simulink model "TestA__03"  (R2015b)
settings: Solver=ode23tb  StartTime=0.0  StopTime=.3  RelTol=1e-3
PreLoadFcn:
  | t1=1;
InitFcn:
  | t_Pref1=0.09; Pref1=10e2;
  | t_Pref2=0.3;   Pref2=3e5;
  | 
  | t_Qmax1=.12; t_Qmax2=t_Qmax1+.01;
  | t_Qref1=0.09; Qref1=7e5;
  | t_Qref2=0.5; Qref2=10e5;
  | 
  | t_Imax1=.2; Imax1=1200;
  | t_Imax2=.4; Imax2=1500;
  | 
  | t_k1=0.25; k1=.8;
  | t_k2=0.35; k2=.2;
  | t_h1=0.45; h1=.9;
  | t_h2=0.55; h2=.5;
  | 
  | Lg=90e-6;
  | l=100e-6; r=2e-3;
  | tff=10e-6;
  | w=2*pi*60;
  | z_lead =966.3602;
  | p_lead =5.6324e+03;
  | Vdc=10000;
  | Vs=690;
undefined symbols (not defined in the file or in its folder): magnitude
libraries: powerlib x43, powerlib_meascontrol x10, simulink x4, simulink_extras x3
settings Model: Creator=Shahed Mortazavian  LastModifiedBy=Masoud
settings DataIOCC: SaveFormat=Array  SignalLoggingSaveFormat=ModelDataLogs
settings OptimizationCC: ExpressionDepthLimit=2147483647
settings DebuggingCC: UnderspecifiedInitializationDetection=Classic  MergeDetectMultiDrivingBlocksExec=none  SolverPrmCheckMsg=warning  FcnCallInpInsideContextMsg=UseLocalSettings  StateNameClashWarn=warning
settings HardwareCC: ProdBitPerPointer=32  ProdLargestAtomicFloat=None  ProdIntDivRoundTo=Undefined  ProdEndianess=Unspecified  ProdWordSize=32  ProdHWDeviceType=32-bit Generic
settings GRTTargetCC: GeneratePreprocessorConditionals=Disable all  CombineOutputUpdateFcns=off  GRTInterface=on
settings ConfigComp: CovModelRefEnable=Off  CovSFcnEnable=off

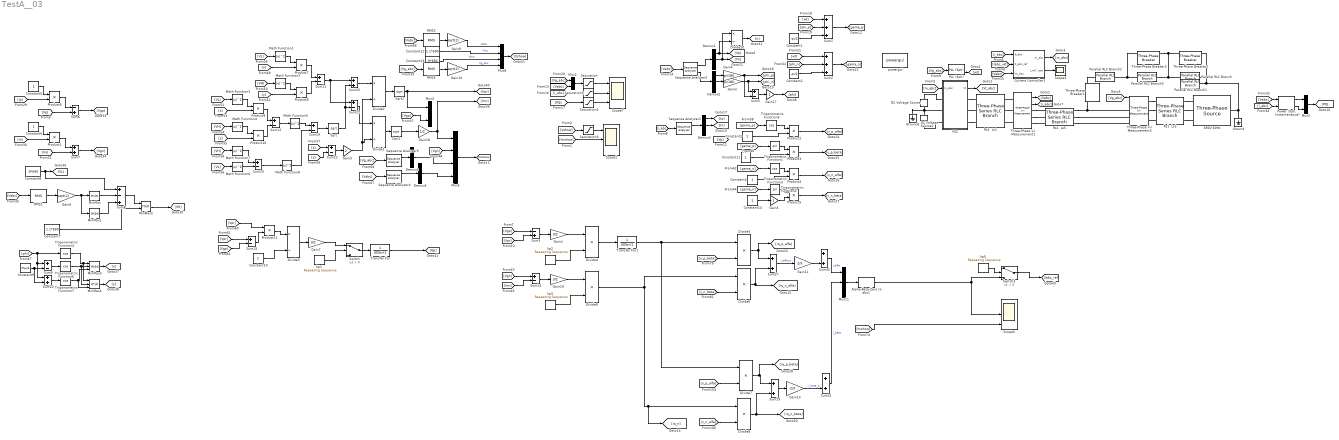
== system TestA__03 ==
  690V 60Hz : powerlib/Electrical Sources/Three-Phase Source  InternalConnection=Yn  VoltagePhases=off  Voltage=Vs*sqrt(3)/sqrt(2)  PhaseAngle=0  Voltage_phases=[25e3 25e3 25e3]/sqrt(3)  PhaseAngles_phases=[0 -120 +120]  Frequency=60  NonIdealSource=on  SpecifyImpedance=off  Resistance=2e-10  Inductance=1e-10  ShortCircuitLevel=100e6  BaseVoltage=25e3  XRratio=7  BusType=swing  Pref=0  Qref=0  Prefabc=[10e3, 10e3, 10e3]  Qrefabc=[0, 0, 0]  Qmin=-inf  Qmax=inf
  Alpha-Beta-Zero to abc1 : powerlib_meascontrol/Transformations/Alpha-Beta-Zero to abc
  Constant1 : Constant  Value=-pi/2
  Constant{3..6,10..11,14} (7 alike) : Constant
  Constant12 : Constant  Value=1.1*690
  Constant13 : Constant  Value=.9*690
  Constant2 : Constant  Value=-pi/2
  Constant7 : Constant  Value=1.1*690
  Constant8 : Constant  Value=.9*690
  Constant9 : Constant  Value=2*pi/3
  Current Controller1 : Subsystem
  DC Voltage Source : powerlib/Electrical Sources/DC Voltage Source  Amplitude=Vdc/2  Measurements=None
  DC Voltage Source1 : powerlib/Electrical Sources/DC Voltage Source  Amplitude=Vdc/2  Measurements=None
  Demux{1..5} (5 alike) : Demux  Outputs=3
  Divide{1..3,20} (4 alike) : Product  Inputs=*/
  Divide{4..9} (6 alike) : Product  Inputs=**
  Gain1 : Gain  Gain=3/2
  Gain10 : Gain  Gain=-2/3
  Gain11 : Gain  Gain=2/3
  Gain16 : Gain  Gain=sqrt(2)
  Gain17 : Gain
  Gain18 : Gain  Gain=1/2
  Gain19 : Gain  Gain=3/2
  Gain2 : Gain  Gain=pi/180
  Gain3 : Gain  Gain=2
  Gain4 : Gain  Gain=pi/180
  Gain5 : Gain  Gain=-1
  Gain6 : Gain  Gain=sqrt(2)
  Gain7 : Gain  Gain=3/2
  Gain9 : Gain  Gain=sqrt(2)
  Ground : powerlib/Elements/Ground  LConnTagsString=a
  Ground1 : powerlib/Elements/Ground  LConnTagsString=a
  Math Function{1..8} (8 alike) : Math  Operator=magnitude^2  SaturateOnIntegerOverflow=on
  MinMax : MinMax
  MinMax1 : MinMax  Function=max
  MinMax2 : MinMax  Inputs=2
  MinMax3 : MinMax  Function=max  Inputs=3
  MinMax4 : MinMax  Inputs=3
  Mux11 : Mux  Inputs=3
  Mux2 : Mux  Inputs=2
  Mux3 : Mux  Inputs=2
  Mux4 : Mux  Inputs=2
  Mux5 : Mux
  Mux8 : Mux
  PLL (3ph) : powerlib_meascontrol/PLL/PLL (3ph)  Fmin=45  Par_Init=[0, 60]  ParK=[180, 3200, 1]  TcD=1e-4  MaxRateChangeFreq=12  FilterCutOffFreq=25  Ts=0  AGC=on
  Parallel RLC Branch : powerlib/Elements/Parallel RLC Branch  LConnTagsString=a  RConnTagsString=__new0  BranchType=R  Resistance=2e-3  Inductance=1e-3  SetiL0=off  InitialCurrent=0  Capacitance=1e-6  Setx0=off  InitialVoltage=0  Measurements=None
  Parallel RLC Branch1 : powerlib/Elements/Parallel RLC Branch  LConnTagsString=a  RConnTagsString=__new0  BranchType=R  Resistance=.02  Inductance=1e-3  SetiL0=off  InitialCurrent=0  Capacitance=1e-6  Setx0=off  InitialVoltage=0  Measurements=None
  Parallel RLC Branch2 : powerlib/Elements/Parallel RLC Branch  LConnTagsString=a  RConnTagsString=__new0  BranchType=R  Resistance=3e-3  Inductance=1e-3  SetiL0=off  InitialCurrent=0  Capacitance=1e-6  Setx0=off  InitialVoltage=0  Measurements=None
  Parallel RLC Branch3 : powerlib/Elements/Parallel RLC Branch  LConnTagsString=a  RConnTagsString=__new0  BranchType=R  Resistance=1e-3  Inductance=1e-3  SetiL0=off  InitialCurrent=0  Capacitance=1e-6  Setx0=off  InitialVoltage=0  Measurements=None
  "Power (3ph, Instantaneous)" : powerlib_meascontrol/Measurements/Power (3ph, Instantaneous)
  Product{1..11} (11 alike) : Product
  RMS1 : powerlib_meascontrol/Measurements/RMS  TrueRMS=on  Freq=60  RMSInit=0  Ts=0
  RMS2 : powerlib_meascontrol/Measurements/RMS  TrueRMS=on  Freq=60  RMSInit=0  Ts=0
  RMS5 : powerlib_meascontrol/Measurements/RMS  TrueRMS=on  Freq=60  RMSInit=0  Ts=0
  Rs1  Ls1 : powerlib/Elements/Three-Phase Series RLC Branch  LConnTagsString=A|B|C  RConnTagsString=A|B|C  BranchType=RL  Resistance=r  Inductance=l  Capacitance=1e-6  Measurements=None
  Rs1  Ls2 : powerlib/Elements/Three-Phase Series RLC Branch  LConnTagsString=A|B|C  RConnTagsString=A|B|C  BranchType=R  Resistance=1e-3  Inductance=l  Capacitance=1e-6  Measurements=None
  Rs1  Ls5 : powerlib/Elements/Three-Phase Series RLC Branch  LConnTagsString=A|B|C  RConnTagsString=A|B|C  BranchType=RL  Resistance=1e-3  Inductance=1/377  Capacitance=1e-6  Measurements=None
  Saturation : Saturate  UpperLimit=1000  LowerLimit=-1000
  Saturation1 : Saturate  UpperLimit=200  LowerLimit=-200
  Saturation2 : Saturate  UpperLimit=2e5  LowerLimit=-1e5
  Saturation3 : Saturate  UpperLimit=800  LowerLimit=400
  Scope2 : Scope  NumInputPorts=3
  Scope3 : Scope
  Scope5 : Scope  NumInputPorts=3
  Scope7 : Scope  NumInputPorts=3
  Sequence Analyzer{1..4} (4 alike) : powerlib_meascontrol/Measurements/Sequence Analyzer  Freq=60  n=1  seq=Positive Negative Zero  InInit=[1, 0]  Ts=0
  Sqrt : Sqrt  SaturateOnIntegerOverflow=on
  Sqrt1 : Sqrt  SaturateOnIntegerOverflow=on
  Sqrt2 : Sqrt  SaturateOnIntegerOverflow=on
  Sum1 : Sum  Inputs=+++
  Sum{7,10,23,27,29..31} (7 alike) : Sum
  Sum{5,9,11..12,14,19..22,24} (10 alike) : Sum  Inputs=+-
  Sum2 : Sum  Inputs=+++
  Sum3 : Sum  Inputs=-+
  Sum6 : Sum  Inputs=-+
  Sum8 : Sum  Inputs=+-+
  Switch : Switch  Criteria=u2 > Threshold
  Switch3 : Switch  Criteria=u2 > Threshold
  Three-Phase V-I Measurement1 : powerlib/Measurements/Three-Phase V-I Measurement  VoltageMeasurement=phase-to-ground  SetLabelV=off  LabelV=Vabc  Vpu=off  VpuLL=off  CurrentMeasurement=yes  SetLabelI=off  LabelI=Iabc  Ipu=off  Pbase=100e6  Vbase=500e3  OutputType=Complex  PhasorSimulation=off  PSBequivalent=0
  Three-Phase V-I Measurement3 : powerlib/Measurements/Three-Phase V-I Measurement  VoltageMeasurement=phase-to-ground  SetLabelV=off  LabelV=Vabc  Vpu=off  VpuLL=off  CurrentMeasurement=yes  SetLabelI=off  LabelI=Iabc  Ipu=off  Pbase=100e6  Vbase=500e3  OutputType=Complex  PhasorSimulation=off  PSBequivalent=0
  Three-Phase Breaker1 : powerlib/Elements/Three-Phase Breaker  InitialState=open  SwitchA=on  SwitchB=on  SwitchC=on  SwitchTimes=[.05 10]  External=off  BreakerResistance=1e-40  SnubberResistance=1e6  SnubberCapacitance=inf  Measurements=None
  Three-Phase Breaker2 : powerlib/Elements/Three-Phase Breaker  InitialState=open  SwitchA=on  SwitchB=on  SwitchC=on  SwitchTimes=.1  External=off  BreakerResistance=1e-40  SnubberResistance=1e6  SnubberCapacitance=inf  Measurements=None
  Three-Phase Breaker3 : powerlib/Elements/Three-Phase Breaker  InitialState=open  SwitchA=on  SwitchB=on  SwitchC=on  SwitchTimes=.15  External=off  BreakerResistance=1e-40  SnubberResistance=1e6  SnubberCapacitance=inf  Measurements=None
  Transfer Fcn : TransferFcn  Denominator=[.005 1]
  Transfer Fcn1 : TransferFcn  Denominator=[.005 1]
  Trigonometric Function1 : Trigonometry
  Trigonometric Function2 : Trigonometry
  Trigonometric Function{3..7} (5 alike) : Trigonometry  Operator=cos
  VSC : Subsystem
  kp1 : simulink/Sources/Repeating Sequence  rep_seq_t=[0 .055 .055+eps 10]  rep_seq_y=[0 0 1 1]
  kp2 : simulink/Sources/Repeating Sequence  rep_seq_t=[0 .055 .055+eps 10]  rep_seq_y=[0 0 1 1]
  kp3 : simulink/Sources/Repeating Sequence  rep_seq_t=[0 .2 .2+eps 10]  rep_seq_y=[0 0 1 1]
  kp5 : simulink/Sources/Repeating Sequence  rep_seq_t=[0 .6 .6+eps 10]  rep_seq_y=[0 0 1 1]
  powergui : powerlib/powergui  Priority=2  SimulationMode=Discrete  SolverType=Tustin  SampleTime=5e-5  frequency=60  SPID=off  DisableSnubberDevices=off  DisableRonSwitches=off  DisableVfSwitches=off  SwTol=0  DisplayEquations=off  Interpol=off  ExternalGateDelay=off  methode=off  Ts=0  FunctionMessages=off  echomessages=off  HookPort=off  EnableUseOfTLC=off  x0status=blocks  frequencyindice=0  Pbase=100e6  ErrMax=1e-4  Iterations=50  UnitsV=kV  UnitsW=MW  buscounter=0  RestoreLinks=warning  ResistiveCurrentMeasurement=off  Frange=[0:2:500]  Ylog=off  Xlog=on  ShowGrid=off  save=off  variable=ZData  structure=Data  ZoomFFT=off  StartTime=.22  cycles=2  DisplayStyle=1  fundamental=60  FreqAxis=off  MaxFrequency=1000  frequencyindicesteady=1  RmsSteady=1  display=off
  wires:
  Three-Phase V-I Measurement1/1 -> [Vabc]
  VSC/1(Vt) -> [Vt_abc]
  [m_abc] -> VSC/1(m_abc)
  Three-Phase V-I Measurement3/1 -> [Vg_abc]
  Three-Phase V-I Measurement1/2 -> [i_abc]
  [Vabc] -> Sequence Analyzer2/1
  [i_abc] -> Current Controller1/1(It_abc)
  [Vabc] -> Current Controller1/3(Vs_abc)
  Current Controller1/1(m_abc) -> [m_abc]
  [Iabc_ref] -> Current Controller1/2(It_abc_ref)
  [Vg_abc] -> PLL (3ph)/1
  PLL (3ph)/2 -> [wt]
  [i_abc] -> Saturation1/1
  [PQ] -> Saturation2/1
  Mux2/1 -> Saturation/1
  [Vabc] -> Mux2/2
  [Vg_abc] -> Mux2/1
  Sequence Analyzer2/1 -> Demux1/1
  Demux1/1 -> Divide20/2, [Vp]
  Demux2/1 -> Gain4/1
  Sequence Analyzer2/2 -> Demux2/1
  Demux2/2 -> Gain2/1
  Demux1/2 -> Divide20/1, [Vn]
  "Power (3ph, Instantaneous)"/1 -> Mux3/1
  "Power (3ph, Instantaneous)"/2 -> Mux3/2
  [Vabc] -> "Power (3ph, Instantaneous)"/1
  [i_abc] -> "Power (3ph, Instantaneous)"/2
  Mux3/1 -> [PQ]
  Gain4/1 -> [phi_p], Sum5/2
  Gain2/1 -> [phi_n], Sum5/1
  [gama_p] -> Trigonometric Function5/1
  Trigonometric Function5/1 -> Product2/1
  Constant3/1 -> Product2/2
  [gama_p] -> Trigonometric Function1/1
  Trigonometric Function1/1 -> Product3/1
  [gama_n] -> Trigonometric Function3/1
  Trigonometric Function3/1 -> Product4/1
  Product4/1 -> [v_n_alfa]
  [gama_n] -> Trigonometric Function2/1
  Trigonometric Function2/1 -> Product5/1
  Product5/1 -> [v_n_beta]
  Constant14/1 -> Gain5/1
  Constant4/1 -> Product4/2
  Gain5/1 -> Product5/2
  Product2/1 -> [v_p_alfa]
  Product3/1 -> [v_p_beta]
  Constant11/1 -> Product3/2
  Sum5/1 -> Gain17/1
  [Vp] -> Sum6/2
  Constant5/1 -> Product6/1
  [i_abc] -> Sequence Analyzer1/1
  Sequence Analyzer1/1 -> Demux3/1
  Demux3/1 -> [Ip]
  Demux3/2 -> [In]
  [Ip] -> Product6/2
  Product6/1 -> Sum6/1
  Sum6/1 -> [Vgp]
  [Vn] -> Sum7/2
  Constant6/1 -> Product1/1
  [In] -> Product1/2
  Product1/1 -> Sum7/1
  Sum7/1 -> [Vgn]
  RMS1/1 -> Gain6/1
  Gain6/1 -> MinMax1/1, MinMax/1
  [Vabc] -> RMS1/1
  Constant8/1 -> Sum8/1, [VL]
  MinMax/1 -> Sum8/2
  MinMax1/1 -> Sum8/3
  Constant7/1 -> MinMax2/2
  Sum8/1 -> MinMax2/1
  Current Controller1/2(I_ref_meas) -> Scope3/1
  MinMax2/1 -> [VH]
  [phi] -> Sum10/1, Sum9/1, Trigonometric Function4/1
  Constant9/1 -> Sum10/2, Sum9/2
  Sum9/1 -> Trigonometric Function6/1
  Sum10/1 -> Trigonometric Function7/1
  Trigonometric Function4/1 -> MinMax4/1, MinMax3/1
  Trigonometric Function6/1 -> MinMax4/2, MinMax3/2
  Trigonometric Function7/1 -> MinMax4/3, MinMax3/3
  MinMax3/1 -> [x]
  MinMax4/1 -> [y]
  [VL] -> Math Function1/1
  Math Function1/1 -> Product7/1
  [x] -> Product7/2
  [VH] -> Math Function2/1
  Math Function2/1 -> Product8/1
  [y] -> Product8/2
  Product7/1 -> Sum11/1
  Product8/1 -> Sum11/2
  [VL] -> Math Function3/1
  Math Function3/1 -> Product9/1
  [x] -> Product9/2
  [VH] -> Math Function4/1
  Math Function4/1 -> Product10/1
  [y] -> Product10/2
  Product9/1 -> Sum12/1
  Product10/1 -> Sum12/2
  Sum12/1 -> Math Function5/1
  Math Function5/1 -> Sum19/1
  [VL] -> Math Function6/1
  [VH] -> Math Function7/1
  Math Function7/1 -> Sum20/1
  Math Function6/1 -> Sum20/2
  Sum20/1 -> Math Function8/1
  Math Function8/1 -> Sum19/2
  Sum19/1 -> Sqrt/1
  Sqrt/1 -> Sum23/2, Sum21/2
  Sum11/1 -> Sum21/1, Sum23/1
  Sum21/1 -> Divide1/1
  [x] -> Sum22/1
  [y] -> Sum22/2
  Sum22/1 -> Gain3/1
  Gain3/1 -> Divide2/2, Divide1/2
  Divide1/1 -> Sqrt1/1
  Sum23/1 -> Divide2/1
  Sqrt2/1 -> [Vpr], Mux4/1
  Divide2/1 -> Sqrt2/1
  [Vpr] -> Product11/1
  [Vpr] -> Sum24/1
  [Vgp] -> Sum24/2
  Sum24/1 -> Product11/2
  Constant10/1 -> Divide3/2
  Product11/1 -> Divide3/1
  Divide3/1 -> Gain7/1
  RMS2/1 -> Gain9/1
  [Vabc] -> RMS2/1
  Gain9/1 -> Mux8/1  "Vabc"
  Constant12/1 -> Mux8/2  "Vup"
  Constant13/1 -> Mux8/3  "Vlow"
  Mux8/1 -> [Vshow]
  [v_p_beta] -> Divide5/2
  Divide5/1 -> [iq_p_alfa], Sum27/1
  Divide6/1 -> [iq_n_alfa], Sum27/2
  [v_n_beta] -> Divide6/2
  Sum27/1 -> Gain11/1  "i_alfa_q"
  Gain10/1 -> Sum31/2  "i_beta_q"
  Sum29/1 -> Gain10/1
  Mux11/1 -> Alpha-Beta-Zero to abc1/1
  Sum30/1 -> Mux11/1  "i_alfa"
  Sum31/1 -> Mux11/2  "I_beta"
  [Vnshow] -> Scope5/3
  [v_p_alfa] -> Divide7/2
  Divide7/1 -> [iq_p_beta], Sum29/1
  Divide8/1 -> Sum29/2, [iq_n_beta]
  [v_n_alfa] -> Divide8/2
  Gain11/1 -> Sum30/2
  [wt] -> Sum1/1
  [phi_p] -> Sum1/2
  Sum1/1 -> [gama_p]
  [wt] -> Sum2/1
  [phi_n] -> Sum2/2
  Sum2/1 -> [gama_n]
  Constant1/1 -> Sum1/3
  Constant2/1 -> Sum2/3
  Alpha-Beta-Zero to abc1/1 -> Scope5/2, Switch3/3
  Switch/1 -> Transfer Fcn/1
  Gain7/1 -> Switch/1
  kp1/1 -> Switch/2
  Divide4/1 -> Transfer Fcn1/1
  RMS5/1 -> Gain16/1
  [Vg_abc] -> RMS5/1
  Gain16/1 -> Mux8/4  "Vg_abc"
  [Vgp] -> Mux4/2
  [Vgn] -> Mux5/2
  Mux5/1 -> [Vnshow]
  Sqrt1/1 -> Gain18/1
  Gain17/1 -> [phi]
  Gain18/1 -> Mux5/1, [Vnr]
  Transfer Fcn/1 -> [Qp]
  kp5/1 -> Switch3/2
  Switch3/1 -> [Iabc_ref]
  [Vg_abc] -> Sequence Analyzer3/1
  Sequence Analyzer3/1 -> Demux4/1
  Demux4/2 -> Mux5/3
  [Vnr] -> Sum14/2
  [Vgn] -> Sum14/1
  Divide9/1 -> [iq_n], Divide8/1, Divide6/1
  Sum14/1 -> Gain19/1
  kp3/1 -> Divide9/2
  [Vabc] -> Sequence Analyzer4/1
  Sequence Analyzer4/1 -> Demux5/1
  Demux5/2 -> Mux5/4
  Gain19/1 -> Divide9/1
  Divide20/1 -> [n]
  [Vnshow] -> Scope2/2
  [Vshow] -> Saturation3/1
  Saturation/1 -> Scope7/1
  Saturation1/1 -> Scope7/2
  Saturation2/1 -> Scope7/3
  Saturation3/1 -> Scope2/1
  [Vpr] -> Sum3/2
  [Vgp] -> Sum3/1
  Sum3/1 -> Gain1/1
  kp2/1 -> Divide4/2
  Gain1/1 -> Divide4/1
  Transfer Fcn1/1 -> Divide7/1, Divide5/1
  connections:
  Three-Phase V-I Measurement1/LConn1 -- Rs1  Ls1/RConn1
  Three-Phase V-I Measurement1/LConn2 -- Rs1  Ls1/RConn2
  Three-Phase V-I Measurement1/LConn3 -- Rs1  Ls1/RConn3
  Parallel RLC Branch/LConn1 -- Parallel RLC Branch3/RConn1 -- Three-Phase Breaker2/LConn1 -- Three-Phase Breaker3/RConn1
  VSC/RConn1 -- Rs1  Ls1/LConn1
  VSC/RConn2 -- Rs1  Ls1/LConn2
  VSC/RConn3 -- Rs1  Ls1/LConn3
  DC Voltage Source/RConn1 -- VSC/LConn1
  DC Voltage Source1/LConn1 -- VSC/LConn3
  Three-Phase V-I Measurement3/LConn1 -- Rs1  Ls2/LConn1
  Three-Phase V-I Measurement3/LConn2 -- Rs1  Ls2/LConn2
  Rs1  Ls2/LConn3 -- Three-Phase V-I Measurement3/LConn3
  Rs1  Ls2/RConn1 -- 690V 60Hz/RConn1
  Rs1  Ls2/RConn2 -- 690V 60Hz/RConn2
  Rs1  Ls2/RConn3 -- 690V 60Hz/RConn3
  Three-Phase V-I Measurement1/RConn1 -- Rs1  Ls5/LConn1
  Three-Phase V-I Measurement1/RConn2 -- Rs1  Ls5/LConn2
  Three-Phase V-I Measurement1/RConn3 -- Rs1  Ls5/LConn3
  DC Voltage Source/LConn1 -- Ground1/LConn1 -- DC Voltage Source1/RConn1 -- VSC/LConn2
  Ground/LConn1 -- Parallel RLC Branch1/RConn1 -- Three-Phase Breaker2/RConn1 -- Parallel RLC Branch/RConn1 -- 690V 60Hz/LConn1
  Rs1  Ls5/RConn1 -- Three-Phase Breaker1/LConn1 -- Three-Phase V-I Measurement3/RConn1
  Rs1  Ls5/RConn2 -- Three-Phase V-I Measurement3/RConn2
  Rs1  Ls5/RConn3 -- Three-Phase V-I Measurement3/RConn3
  Parallel RLC Branch2/LConn1 -- Three-Phase Breaker1/RConn1
  Parallel RLC Branch3/LConn1 -- Three-Phase Breaker3/LConn1 -- Parallel RLC Branch2/RConn1

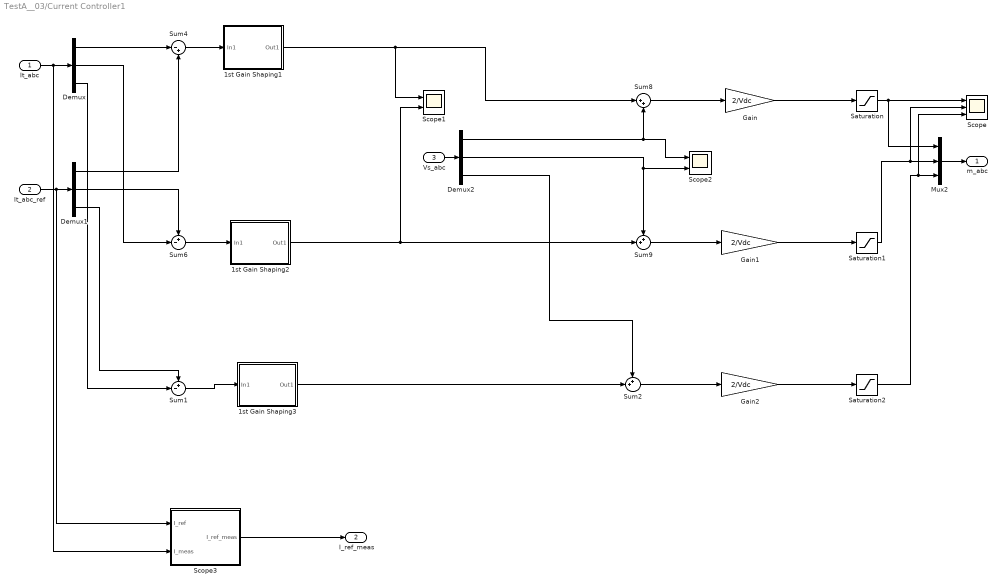
== system TestA__03/Current Controller1 ==
  It_abc : Inport
  It_abc_ref : Inport  Port=2
  Vs_abc : Inport  Port=3
  1st Gain Shaping1 : Subsystem
  1st Gain Shaping2 : Subsystem
  1st Gain Shaping3 : Subsystem
  Demux : Demux  Outputs=3
  Demux1 : Demux  Outputs=3
  Demux2 : Demux  Outputs=3
  Gain : Gain  Gain=2/Vdc
  Gain1 : Gain  Gain=2/Vdc
  Gain2 : Gain  Gain=2/Vdc
  Mux2 : Mux  Inputs=3
  Saturation : Saturate  UpperLimit=1  LowerLimit=-1
  Saturation1 : Saturate  UpperLimit=1  LowerLimit=-1
  Saturation2 : Saturate  UpperLimit=1  LowerLimit=-1
  Scope : Scope  NumInputPorts=3
  Scope1 : Scope  NumInputPorts=2
  Scope2 : Scope  NumInputPorts=2
  Scope3 : Subsystem
  Sum1 : Sum  Inputs=+-|
  Sum2 : Sum  Inputs=++|
  Sum4 : Sum  Inputs=|-+
  Sum6 : Sum  Inputs=+-|
  Sum8 : Sum  Inputs=|++
  Sum9 : Sum  Inputs=++|
  m_abc : Outport
  I_ref_meas : Outport  Port=2
  wires:
  Demux2/1 -> Scope2/1, Sum8/2
  Demux2/2 -> Scope2/2, Sum9/1
  Sum6/1 -> 1st Gain Shaping2/1(In1)
  It_abc/1 -> Scope3/2(I_meas), Demux/1
  It_abc_ref/1 -> Scope3/1(I_ref), Demux1/1
  Vs_abc/1 -> Demux2/1
  Sum8/1 -> Gain/1
  Sum9/1 -> Gain1/1
  Mux2/1 -> m_abc/1
  Gain/1 -> Saturation/1
  Gain1/1 -> Saturation1/1
  Saturation2/1 -> Scope/3, Mux2/3
  Saturation/1 -> Scope/1, Mux2/1
  Saturation1/1 -> Mux2/2, Scope/2
  Demux1/1 -> Sum4/2
  Demux/1 -> Sum4/1
  Sum4/1 -> 1st Gain Shaping1/1(In1)
  Demux1/2 -> Sum6/1
  Demux/2 -> Sum6/2
  Demux1/3 -> Sum1/1
  Demux/3 -> Sum1/2
  Sum1/1 -> 1st Gain Shaping3/1(In1)
  Gain2/1 -> Saturation2/1
  Sum2/1 -> Gain2/1
  Demux2/3 -> Sum2/1
  1st Gain Shaping2/1(Out1) -> Scope1/2, Sum9/2
  1st Gain Shaping3/1(Out1) -> Sum2/2
  1st Gain Shaping1/1(Out1) -> Scope1/1, Sum8/1
  Scope3/1(I_ref_meas) -> I_ref_meas/1

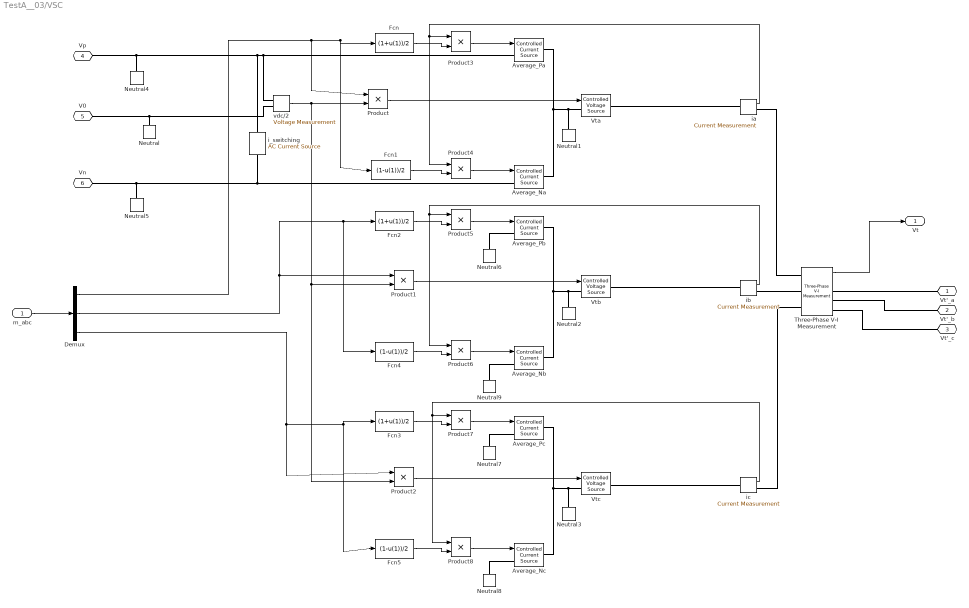
== system TestA__03/VSC ==
  m_abc : Inport
  Average_Na : powerlib/Electrical Sources/Controlled Current Source  Initialize=on  Source_Type=AC  Amplitude=0  Phase=0  Frequency=0  Measurements=None
  Average_Nb : powerlib/Electrical Sources/Controlled Current Source  Initialize=on  Source_Type=AC  Amplitude=0  Phase=0  Frequency=0  Measurements=None
  Average_Nc : powerlib/Electrical Sources/Controlled Current Source  Initialize=on  Source_Type=AC  Amplitude=0  Phase=0  Frequency=0  Measurements=None
  Average_Pa : powerlib/Electrical Sources/Controlled Current Source  Initialize=on  Source_Type=AC  Amplitude=0  Phase=0  Frequency=0  Measurements=None
  Average_Pb : powerlib/Electrical Sources/Controlled Current Source  Initialize=on  Source_Type=AC  Amplitude=0  Phase=0  Frequency=0  Measurements=None
  Average_Pc : powerlib/Electrical Sources/Controlled Current Source  Initialize=on  Source_Type=AC  Amplitude=0  Phase=0  Frequency=0  Measurements=None
  Demux : Demux  Outputs=3
  Fcn : Fcn  Expr=(1+u(1))/2
  Fcn1 : Fcn  Expr=(1-u(1))/2
  Fcn2 : Fcn  Expr=(1+u(1))/2
  Fcn3 : Fcn  Expr=(1+u(1))/2
  Fcn4 : Fcn  Expr=(1-u(1))/2
  Fcn5 : Fcn  Expr=(1-u(1))/2
  Neutral{,1..3} (4 alike) : powerlib/Elements/Neutral  LConnTagsString=a  NodeNumber=10
  Neutral4 : powerlib/Elements/Neutral  LConnTagsString=a  NodeNumber=11
  Neutral5 : powerlib/Elements/Neutral  LConnTagsString=a  NodeNumber=12
  Neutral6 : powerlib/Elements/Neutral  LConnTagsString=a  NodeNumber=11
  Neutral7 : powerlib/Elements/Neutral  LConnTagsString=a  NodeNumber=11
  Neutral8 : powerlib/Elements/Neutral  LConnTagsString=a  NodeNumber=12
  Neutral9 : powerlib/Elements/Neutral  LConnTagsString=a  NodeNumber=12
  Product{,1..8} (9 alike) : Product  RndMeth=Zero
  Three-Phase V-I Measurement : powerlib/Measurements/Three-Phase V-I Measurement  VoltageMeasurement=phase-to-ground  SetLabelV=off  LabelV=Vabc  Vpu=off  VpuLL=off  CurrentMeasurement=yes  SetLabelI=off  LabelI=Iabc  Ipu=off  Pbase=100e6  Vbase=500e3  OutputType=Complex  PhasorSimulation=off  PSBequivalent=0
  Vta : powerlib/Electrical Sources/Controlled Voltage Source  Initialize=on  Source_Type=AC  Amplitude=0  Phase=0  Frequency=0  Measurements=None
  Vtb : powerlib/Electrical Sources/Controlled Voltage Source  Initialize=on  Source_Type=AC  Amplitude=0  Phase=0  Frequency=0  Measurements=None
  Vtc : powerlib/Electrical Sources/Controlled Voltage Source  Initialize=on  Source_Type=AC  Amplitude=0  Phase=0  Frequency=0  Measurements=None
  i_switching : powerlib/Electrical Sources/AC Current Source  Amplitude=1  Phase=0  Frequency=0  SampleTime=0  Measurements=None
  ia : powerlib/Measurements/Current Measurement  PhasorSimulation=off  OutputType=Complex  PSBequivalent=0
  ib : powerlib/Measurements/Current Measurement  PhasorSimulation=off  OutputType=Complex  PSBequivalent=0
  ic : powerlib/Measurements/Current Measurement  PhasorSimulation=off  OutputType=Complex  PSBequivalent=0
  vdc/2 : powerlib/Measurements/Voltage Measurement  PhasorSimulation=off  OutputType=Complex  PSBequivalent=0
  Vt'_a : PMIOPort  Port=1  Side=Right
  Vt'_b : PMIOPort  Port=2  Side=Right
  Vt'_c : PMIOPort  Port=3  Side=Right
  Vp : PMIOPort  Port=4  Side=Left
  V0 : PMIOPort  Port=5  Side=Left
  Vn : PMIOPort  Port=6  Side=Left
  Vt : Outport
  wires:
  Fcn1/1 -> Product4/2
  Fcn2/1 -> Product5/2
  Fcn4/1 -> Product6/2
  Fcn3/1 -> Product7/2
  Fcn5/1 -> Product8/2
  Demux/1 -> Fcn/1, Fcn1/1, Product/1
  Demux/2 -> Fcn2/1, Fcn4/1, Product1/1
  Demux/3 -> Fcn3/1, Fcn5/1, Product2/1
  vdc/2/1 -> Product/2, Product1/2, Product2/2
  Product/1 -> Vta/1
  Product1/1 -> Vtb/1
  Product2/1 -> Vtc/1
  Product3/1 -> Average_Pa/1
  Fcn/1 -> Product3/2
  Product4/1 -> Average_Na/1
  Product5/1 -> Average_Pb/1
  Product7/1 -> Average_Pc/1
  Product8/1 -> Average_Nc/1
  ia/1 -> Product3/1, Product4/1
  ib/1 -> Product5/1, Product6/1
  ic/1 -> Product7/1, Product8/1
  Product6/1 -> Average_Nb/1
  m_abc/1 -> Demux/1
  Three-Phase V-I Measurement/1 -> Vt/1
  connections:
  Vn/RConn1 -- i_switching/RConn1 -- Average_Na/LConn1 -- Neutral5/LConn1
  Vp/RConn1 -- vdc/2/LConn1 -- Average_Pa/LConn1 -- i_switching/LConn1 -- Neutral4/LConn1
  Vta/RConn1 -- ia/LConn1
  Vtb/RConn1 -- ib/LConn1
  Vtc/RConn1 -- ic/LConn1
  Average_Pb/RConn1 -- Average_Nb/RConn1 -- Vtb/LConn1 -- Neutral2/LConn1
  Three-Phase V-I Measurement/LConn1 -- ia/RConn1
  Three-Phase V-I Measurement/LConn2 -- ib/RConn1
  Three-Phase V-I Measurement/LConn3 -- ic/RConn1
  Average_Pa/RConn1 -- Average_Na/RConn1 -- Vta/LConn1 -- Neutral1/LConn1
  Average_Pc/RConn1 -- Average_Nc/RConn1 -- Vtc/LConn1 -- Neutral3/LConn1
  V0/RConn1 -- vdc/2/LConn2 -- Neutral/LConn1
  Neutral6/LConn1 -- Average_Pb/LConn1
  Neutral7/LConn1 -- Average_Pc/LConn1
  Neutral8/LConn1 -- Average_Nc/LConn1
  Neutral9/LConn1 -- Average_Nb/LConn1
  Vt'_a/RConn1 -- Three-Phase V-I Measurement/RConn1
  Three-Phase V-I Measurement/RConn2 -- Vt'_b/RConn1
  Three-Phase V-I Measurement/RConn3 -- Vt'_c/RConn1

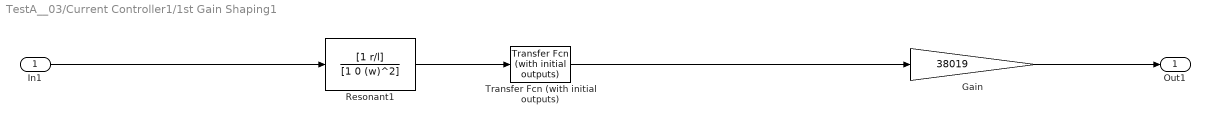
== system TestA__03/Current Controller1/1st Gain Shaping1 ==
  In1 : Inport
  Gain : Gain  Gain=38019
  Resonant1 : TransferFcn  Numerator=[1 r/l]  Denominator=[1 0 (w)^2]
  Transfer Fcn (with initial outputs) : simulink_extras/Additional Linear/Transfer Fcn (with initial outputs)  N=[1 5205]  D=[1 30340]  Y0=0  U0=0
  Out1 : Outport
  wires:
  Resonant1/1 -> Transfer Fcn (with initial outputs)/1
  In1/1 -> Resonant1/1
  Gain/1 -> Out1/1
  Transfer Fcn (with initial outputs)/1 -> Gain/1

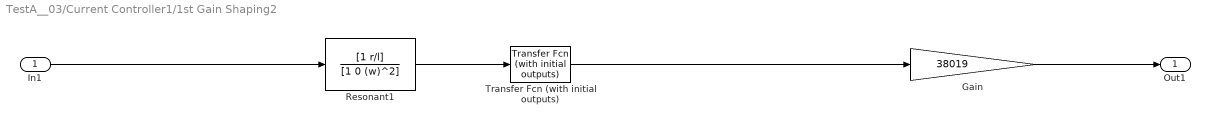
== system TestA__03/Current Controller1/1st Gain Shaping2 ==
  In1 : Inport
  Gain : Gain  Gain=38019
  Resonant1 : TransferFcn  Numerator=[1 r/l]  Denominator=[1 0 (w)^2]
  Transfer Fcn (with initial outputs) : simulink_extras/Additional Linear/Transfer Fcn (with initial outputs)  N=[1 5205]  D=[1 30340]  Y0=0  U0=0
  Out1 : Outport
  wires:
  Transfer Fcn (with initial outputs)/1 -> Gain/1
  Gain/1 -> Out1/1
  In1/1 -> Resonant1/1
  Resonant1/1 -> Transfer Fcn (with initial outputs)/1

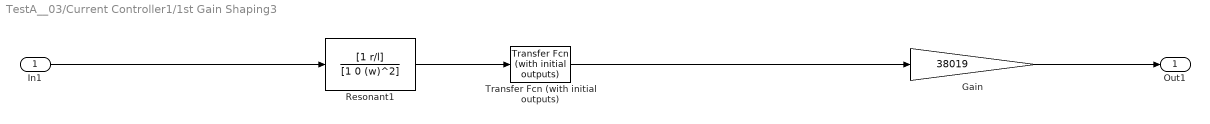
== system TestA__03/Current Controller1/1st Gain Shaping3 ==
  In1 : Inport
  Gain : Gain  Gain=38019
  Resonant1 : TransferFcn  Numerator=[1 r/l]  Denominator=[1 0 (w)^2]
  Transfer Fcn (with initial outputs) : simulink_extras/Additional Linear/Transfer Fcn (with initial outputs)  N=[1 5205]  D=[1 30340]  Y0=0  U0=0
  Out1 : Outport
  wires:
  Resonant1/1 -> Transfer Fcn (with initial outputs)/1
  In1/1 -> Resonant1/1
  Gain/1 -> Out1/1
  Transfer Fcn (with initial outputs)/1 -> Gain/1

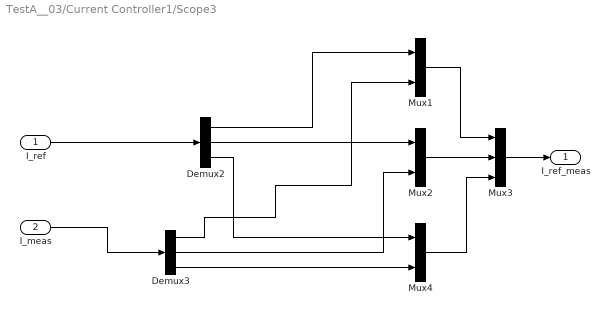
== system TestA__03/Current Controller1/Scope3 ==
  I_ref : Inport
  I_meas : Inport  Port=2
  Demux2 : Demux  Outputs=3
  Demux3 : Demux  Outputs=3
  Mux1 : Mux  Inputs=2
  Mux2 : Mux  Inputs=2
  Mux3 : Mux  Inputs=3
  Mux4 : Mux  Inputs=2
  I_ref_meas : Outport
  wires:
  I_meas/1 -> Demux3/1
  I_ref/1 -> Demux2/1
  Demux2/1 -> Mux1/1
  Demux3/1 -> Mux1/2
  Mux1/1 -> Mux3/1
  Demux2/2 -> Mux2/1
  Demux3/2 -> Mux2/2
  Mux2/1 -> Mux3/2
  Demux2/3 -> Mux4/1
  Demux3/3 -> Mux4/2
  Mux4/1 -> Mux3/3
  Mux3/1 -> I_ref_meas/1
